simulink model "EMR_WindTurbine_Final"  (R2022b)
settings: Solver=VariableStepAuto  StartTime=0.0  StopTime=10.0  RelTol=1e-3
values from neighbouring files (symbols this model uses):
  b = 15    [Init_Celc.m]
  cmaxfit = -4.70546620480099*(10.^-8)*temp.^4+	3.49662102291610*(10.^-6)*temp.^3 +	0.00209286380926111*temp.^2	-0.0176104377910828*temp+	0.0300191236909972    [Init_Celc.m]
  f = 0.001    [Init_Celc.m]
  J = 0.0015    [Init_Celc.m]
  kr = 1    [Init_Celc.m]
  Ktm = 1.5692    [Init_Celc.m]
  Lr = 0.2395    [Init_Celc.m]
  Ls = 0.256    [Init_Celc.m]
  Msr = 0.236    [Init_Celc.m]
  P = 2    [Init_Celc.m]
  r = 0.75    [Init_Celc.m]
  rho = 1.20    (= 1.2)    [Init_Celc.m]
  Rr = 1.09    [Init_Celc.m]
  Rs = 3.36    [Init_Celc.m]
  s = pi*r.^2    [Init_Celc.m]
  temp = (1:vit_syn/40:vit_syn)    [Init_Celc.m]
  UDC = 620    [Init_Celc.m]
  vf = 230/(2*pi*50)    (= 0.732112738223)    [Init_Celc.m]
settings Model: Creator=habayah  LastModifiedBy=ZinouAb
settings ModelReferenceCC: EnableRefExpFcnMdlSchedulingChecks=on

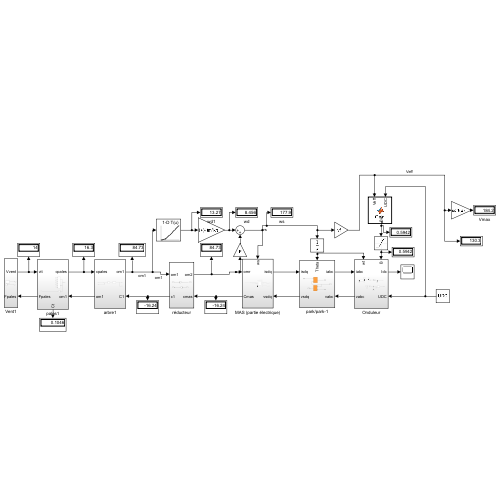
[thumbnail: Simulink's stored preview of the top-level diagram]
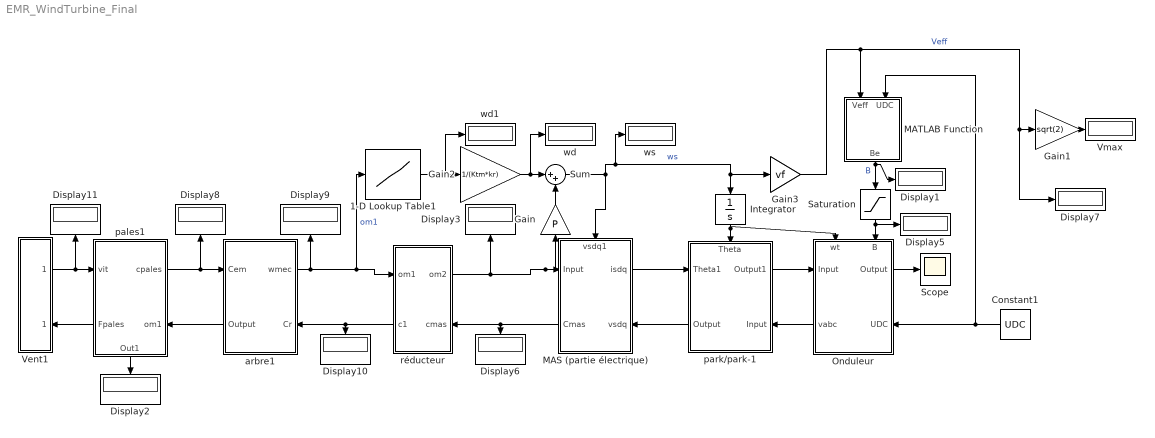
== system EMR_WindTurbine_Final ==
  1-D Lookup Table1 : Lookup_n-D  NumberOfTableDimensions=1  BreakpointsForDimension1=temp  Table=cmaxfit  InternalRulePriority=Speed  RndMeth=Simplest
  Constant1 : Constant  Value=UDC
  Display{1..3,5..11} (10 alike) : Display
  Gain : Gain  Gain=P
  Gain1 : Gain  Gain=sqrt(2)
  Gain2 : Gain  Gain=1/(Ktm*kr)
  Gain3 : Gain  Gain=vf
  Integrator : Integrator
  MAS (partie électrique) : Subsystem
      settings: PortSchema="{\"entries\":[{\"content\":{\"sides\":[{\"content\":{\"connectorIds\":[\"Out2\",\"In1\"]},\"type\":\"ConnectorPlacement.EquallySpacedRectSide\",\"uuid\":\"2ecec5eb-5bb6-4f05-bbbb-1a51ae98f814\"},{\"content\":{\"connectorIds\":[\"In3\",\"Out1\"],\"side\":\"RIGHT\"},\"type\":\"ConnectorPlacement.EquallySpacedRectSide\",\"uuid\":\"ddc3d36f-31b1-43d5-b617-6997f76d08f1\"},{\"content\":{\"connectorIds\":[\"In2\"],\"side\":\"TOP\"},\"type\":\"ConnectorPlacement.EquallySpacedRectSide\",\"uuid\":\"42603242-cda1-4bb2-8cac-1b3409f39577\"}]},\"type\":\"ConnectorPlacement.EquallySpacedConnector\",\"uuid\":\"febb8687-16a8-4638-bd43-9ebf443fd4bd\"}],\"packageUris\":[\"http://schema.mathworks.com/mf0/Connector/R2020b\"],\"version\":\"1.0\"}"
  MATLAB Function : MATLAB Function  TreatAsAtomicUnit=on
  Onduleur : Subsystem
      settings: PortSchema="{\"entries\":[{\"content\":{\"sides\":[{\"content\":{\"connectorIds\":[\"In1\",\"Out2\"]},\"type\":\"ConnectorPlacement.EquallySpacedRectSide\",\"uuid\":\"b96697a1-7390-4a4c-a090-1d4840f94579\"},{\"content\":{\"connectorIds\":[\"Out1\",\"In4\"],\"side\":\"RIGHT\"},\"type\":\"ConnectorPlacement.EquallySpacedRectSide\",\"uuid\":\"06d1d8c6-d481-421b-9786-6ed8bea33fb5\"},{\"content\":{\"connectorIds\":[\"In2\",\"In3\"],\"side\":\"TOP\"},\"type\":\"ConnectorPlacement.EquallySpacedRectSide\",\"uuid\":\"2e081ee8-1238-4450-99c4-3d0e60d3e391\"}]},\"type\":\"ConnectorPlacement.EquallySpacedConnector\",\"uuid\":\"e9990dc2-fc0c-4c65-980c-f90091d8c920\"}],\"packageUris\":[\"http://schema.mathworks.com/mf0/Connector/R2020b\"],\"version\":\"1.0\"}"
  Saturation : Saturate  UpperLimit=1  LowerLimit=0
  Scope : Scope
  Sum : Sum  Inputs=|++
  Vent1 : Subsystem
      settings: PortSchema="{\"entries\":[{\"content\":{\"sides\":[{\"content\":{\"connectorIds\":[]},\"type\":\"ConnectorPlacement.EquallySpacedRectSide\",\"uuid\":\"be9e5db0-62db-41cd-9655-d6d790779573\"},{\"content\":{\"connectorIds\":[\"Out1\",\"In1\"],\"side\":\"RIGHT\"},\"type\":\"ConnectorPlacement.EquallySpacedRectSide\",\"uuid\":\"b5e788b3-1e5f-4899-a162-7a564b67bc63\"},{\"content\":{\"connectorIds\":[],\"side\":\"TOP\"},\"type\":\"ConnectorPlacement.EquallySpacedRectSide\",\"uuid\":\"cac5ef03-1794-4810-a86f-81d9785b0908\"}]},\"type\":\"ConnectorPlacement.EquallySpacedConnector\",\"uuid\":\"fdefeacd-144d-477b-b7c5-141053c244e1\"}],\"packageUris\":[\"http://schema.mathworks.com/mf0/Connector/R2020b\"],\"version\":\"1.0\"}"
  Vmax : Display
  arbre1 : Subsystem
      settings: PortSchema="{\"entries\":[{\"content\":{\"sides\":[{\"content\":{\"connectorIds\":[\"In1\",\"Out2\"]},\"type\":\"ConnectorPlacement.EquallySpacedRectSide\",\"uuid\":\"b8908f99-787f-4ebd-a8c4-361ef654133e\"},{\"content\":{\"connectorIds\":[\"Out1\",\"In2\"],\"side\":\"RIGHT\"},\"type\":\"ConnectorPlacement.EquallySpacedRectSide\",\"uuid\":\"e7049b46-0747-4182-8580-458ffa90f1c3\"},{\"content\":{\"connectorIds\":[],\"side\":\"TOP\"},\"type\":\"ConnectorPlacement.EquallySpacedRectSide\",\"uuid\":\"013bc89f-8670-489b-af07-681a8894793a\"}]},\"type\":\"ConnectorPlacement.EquallySpacedConnector\",\"uuid\":\"dba8a148-0e4d-4308-b676-65e370746724\"}],\"packageUris\":[\"http://schema.mathworks.com/mf0/Connector/R2020b\"],\"version\":\"1.0\"}"
  pales1 : Subsystem
      settings: PortSchema="{\"entries\":[{\"content\":{\"sides\":[{\"content\":{\"connectorIds\":[\"In1\",\"Out3\"]},\"type\":\"ConnectorPlacement.EquallySpacedRectSide\",\"uuid\":\"2ecec5eb-5bb6-4f05-bbbb-1a51ae98f814\"},{\"content\":{\"connectorIds\":[\"Out1\",\"In2\"],\"side\":\"RIGHT\"},\"type\":\"ConnectorPlacement.EquallySpacedRectSide\",\"uuid\":\"ddc3d36f-31b1-43d5-b617-6997f76d08f1\"},{\"content\":{\"connectorIds\":[],\"side\":\"TOP\"},\"type\":\"ConnectorPlacement.EquallySpacedRectSide\",\"uuid\":\"42603242-cda1-4bb2-8cac-1b3409f39577\"},{\"content\":{\"connectorIds\":[\"Out2\"],\"side\":\"BOTTOM\"},\"type\":\"ConnectorPlacement.EquallySpacedRectSide\",\"uuid\":\"35b11503-f988-4bb4-a280-dcf5d49d8570\"}]},\"type\":\"ConnectorPlacement.EquallySpacedConnector\",\"uuid\":\"febb8687-16a8-4638-bd43-9ebf443fd4bd\"}],\"packageUris\":[\"http://schema.mathworks.com/mf0/Connector/R2020b\"],\"version\":\"1.0\"}"
  park/park-1 : Subsystem
      settings: PortSchema="{\"entries\":[{\"content\":{\"sides\":[{\"content\":{\"connectorIds\":[\"In1\",\"Out2\"]},\"type\":\"ConnectorPlacement.EquallySpacedRectSide\",\"uuid\":\"83ad06b1-0178-473a-86b5-0d897bfdf029\"},{\"content\":{\"connectorIds\":[\"Out1\",\"In3\"],\"side\":\"RIGHT\"},\"type\":\"ConnectorPlacement.EquallySpacedRectSide\",\"uuid\":\"370b5efa-4dd6-4b26-a8f3-51e0a3b4d610\"},{\"content\":{\"connectorIds\":[\"In2\"],\"side\":\"TOP\"},\"type\":\"ConnectorPlacement.EquallySpacedRectSide\",\"uuid\":\"4ed8d0b1-afea-41b0-b5a1-8f5ae24d8944\"},{\"content\":{\"connectorIds\":[],\"side\":\"BOTTOM\"},\"type\":\"ConnectorPlacement.EquallySpacedRectSide\",\"uuid\":\"28d6add2-f293-47f7-8dcb-eb46b3627242\"}]},\"type\":\"ConnectorPlacement.EquallySpacedConnector\",\"uuid\":\"0d95acdc-2677-48aa-afd9-0dc380a25251\"}],\"packageUris\":[\"http://schema.mathworks.com/mf0/Connector/R2020b\"],\"version\":\"1.0\"}"
  réducteur : Subsystem
      settings: PortSchema="{\"entries\":[{\"content\":{\"sides\":[{\"content\":{\"connectorIds\":[\"In1\",\"Out2\"]},\"type\":\"ConnectorPlacement.EquallySpacedRectSide\",\"uuid\":\"2ecec5eb-5bb6-4f05-bbbb-1a51ae98f814\"},{\"content\":{\"connectorIds\":[\"Out1\",\"In2\"],\"side\":\"RIGHT\"},\"type\":\"ConnectorPlacement.EquallySpacedRectSide\",\"uuid\":\"ddc3d36f-31b1-43d5-b617-6997f76d08f1\"},{\"content\":{\"connectorIds\":[],\"side\":\"TOP\"},\"type\":\"ConnectorPlacement.EquallySpacedRectSide\",\"uuid\":\"42603242-cda1-4bb2-8cac-1b3409f39577\"}]},\"type\":\"ConnectorPlacement.EquallySpacedConnector\",\"uuid\":\"febb8687-16a8-4638-bd43-9ebf443fd4bd\"}],\"packageUris\":[\"http://schema.mathworks.com/mf0/Connector/R2020b\"],\"version\":\"1.0\"}"
  wd : Display
  wd1 : Display
  ws : Display
  wires:
  réducteur/1(om2) -> Display3/1, MAS (partie électrique)/3(Input), Gain/1
  MAS (partie électrique)/1(Cmas) -> Display6/1, réducteur/2(cmas)
  MAS (partie électrique)/2(isdq) -> park/park-1/1(Theta1)
  park/park-1/2(Output) -> MAS (partie électrique)/1(vsdq)
  Gain/1 -> Sum/2
  Integrator/1 -> Onduleur/2(wt), park/park-1/2(Theta)
  Gain2/1 -> wd/1, Sum/1
  Vent1/1(Out1) -> Display11/1, pales1/1(vit)
  réducteur/2(c1) -> arbre1/2(Cr), Display10/1
  pales1/1(cpales) -> arbre1/1(Cem), Display8/1
  arbre1/1(wmec) -> réducteur/1(om1), 1-D Lookup Table1/1, Display9/1  "om1"
  arbre1/2(Output) -> pales1/2(om1)
  pales1/3(Fpales) -> Vent1/1(In1)
  Sum/1 -> MAS (partie électrique)/2(vsdq1), ws/1, Integrator/1, Gain3/1  "ws"
  Gain1/1 -> Vmax/1
  Saturation/1 -> Onduleur/3(B), Display5/1
  Gain3/1 -> Display7/1, Gain1/1, MATLAB Function/1(Veff)  "Veff"
  MATLAB Function/1(Be) -> Display1/1, Saturation/1  "B"
  Constant1/1 -> Onduleur/4(UDC), MATLAB Function/2(UDC)
  Onduleur/2(vabc) -> park/park-1/3(Input)
  park/park-1/1(Output1) -> Onduleur/1(Input)
  Onduleur/1(Output) -> Scope/1
  pales1/2(Out1) -> Display2/1
  1-D Lookup Table1/1 -> wd1/1, Gain2/1

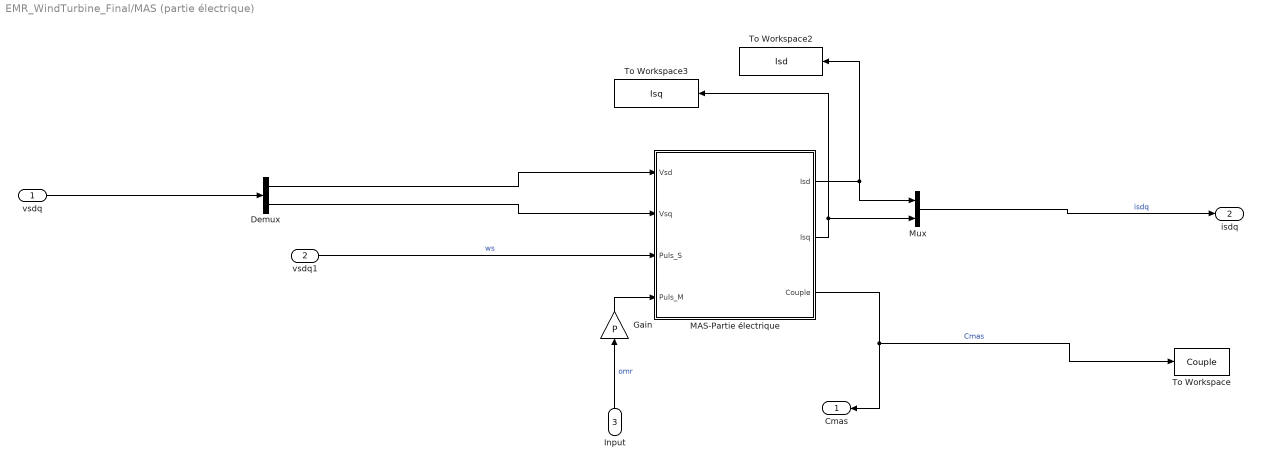
== system EMR_WindTurbine_Final/MAS (partie électrique) ==
  vsdq : Inport
  vsdq1 : Inport  Port=2
  Input : Inport  Port=3
  Demux : Demux  Outputs=2
  Gain : Gain  Gain=P
  MAS-Partie électrique : Subsystem
  Mux : Mux  Inputs=2
  To Workspace : ToWorkspace  VariableName=Couple  SampleTime=-1
      settings: Save2DSignal=2-D array (concatenate along first dimension)
  To Workspace2 : ToWorkspace  VariableName=Isd  SaveFormat=Timeseries  SampleTime=-1
  To Workspace3 : ToWorkspace  VariableName=Isq  SaveFormat=Timeseries  SampleTime=-1
  Cmas : Outport
  isdq : Outport  Port=2
  wires:
  MAS-Partie électrique/2(Isq) -> Mux/2, To Workspace3/1
  MAS-Partie électrique/3(Couple) -> Cmas/1, To Workspace/1  "Cmas"
  Demux/2 -> MAS-Partie électrique/2(Vsq)
  MAS-Partie électrique/1(Isd) -> Mux/1, To Workspace2/1
  Gain/1 -> MAS-Partie électrique/4(Puls_M)
  Input/1 -> Gain/1  "omr"
  Demux/1 -> MAS-Partie électrique/1(Vsd)
  Mux/1 -> isdq/1  "isdq"
  vsdq/1 -> Demux/1
  vsdq1/1 -> MAS-Partie électrique/3(Puls_S)  "ws"

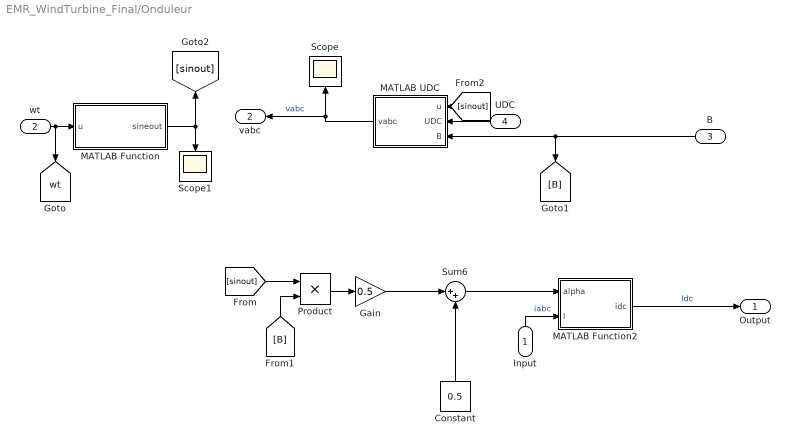
== system EMR_WindTurbine_Final/Onduleur ==
  Input : Inport
  wt : Inport  Port=2
  B : Inport  Port=3
  UDC : Inport  Port=4
  Constant : Constant  Value=0.5
  Gain : Gain  Gain=0.5
  MATLAB Function : MATLAB Function  TreatAsAtomicUnit=on
  MATLAB Function2 : MATLAB Function  TreatAsAtomicUnit=on
  MATLAB UDC : MATLAB Function  TreatAsAtomicUnit=on
  Product : Product
  Scope : Scope
  Scope1 : Scope
  Sum6 : Sum  Inputs=|++
  Output : Outport
  vabc : Outport  Port=2
  tag scope: wt=global
  wires:
  MATLAB Function/1(sineout) -> Scope1/1, [sinout]
  wt/1 -> MATLAB Function/1(u), [wt]
  MATLAB UDC/1(vabc) -> Scope/1, vabc/1  "vabc"
  B/1 -> MATLAB UDC/3(B), [B]
  UDC/1 -> MATLAB UDC/2(UDC)
  [sinout] -> Product/1
  [B] -> Product/2
  Product/1 -> Gain/1
  Sum6/1 -> MATLAB Function2/1(alpha)
  Constant/1 -> Sum6/2
  Input/1 -> MATLAB Function2/2(I)  "iabc"
  MATLAB Function2/1(idc) -> Output/1  "Idc"
  Gain/1 -> Sum6/1
  [sinout] -> MATLAB UDC/1(u)

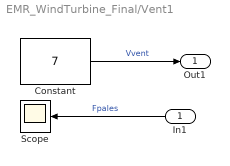
== system EMR_WindTurbine_Final/Vent1 ==
  In1 : Inport
  Constant : Constant  Value=7
  Scope : Scope
  Out1 : Outport
  wires:
  In1/1 -> Scope/1  "Fpales"
  Constant/1 -> Out1/1  "Vvent"

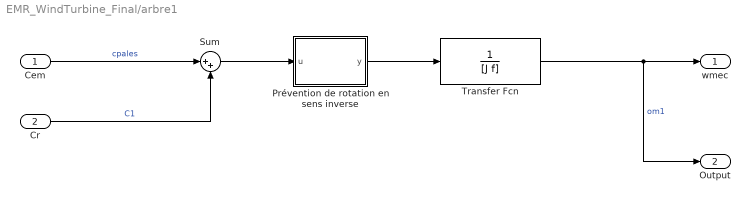
== system EMR_WindTurbine_Final/arbre1 ==
  Cem : Inport
  Cr : Inport  Port=2
  Prévention de rotation en sens inverse : MATLAB Function  TreatAsAtomicUnit=on
  Sum : Sum  Inputs=|++
  Transfer Fcn : TransferFcn  Denominator=[J f]
  wmec : Outport
  Output : Outport  Port=2
  wires:
  Cem/1 -> Sum/1  "cpales"
  Sum/1 -> Prévention de rotation en sens inverse/1(u)
  Cr/1 -> Sum/2  "C1"
  Transfer Fcn/1 -> Output/1, wmec/1  "om1"
  Prévention de rotation en sens inverse/1(y) -> Transfer Fcn/1

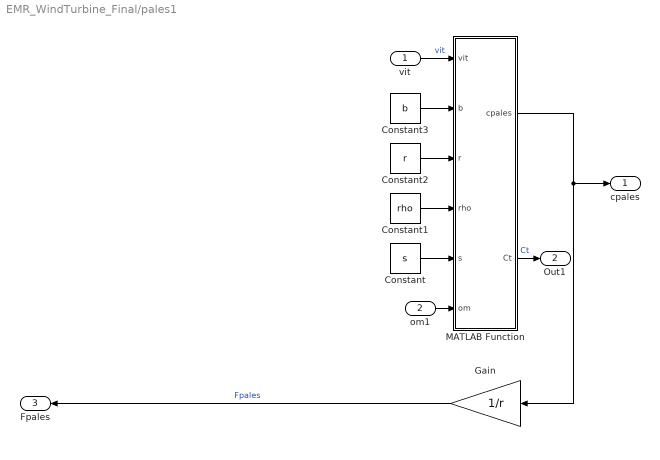
== system EMR_WindTurbine_Final/pales1 ==
  vit : Inport
  om1 : Inport  Port=2
  Constant : Constant  Value=s
  Constant1 : Constant  Value=rho
  Constant2 : Constant  Value=r
  Constant3 : Constant  Value=b
  Gain : Gain  Gain=1/r
  MATLAB Function : MATLAB Function  TreatAsAtomicUnit=on
  cpales : Outport
  Out1 : Outport  Port=2
  Fpales : Outport  Port=3
  wires:
  vit/1 -> MATLAB Function/1(vit)  "vit"
  om1/1 -> MATLAB Function/6(om)
  Constant2/1 -> MATLAB Function/3(r)
  MATLAB Function/1(cpales) -> Gain/1, cpales/1
  Gain/1 -> Fpales/1  "Fpales"
  Constant/1 -> MATLAB Function/5(s)
  Constant1/1 -> MATLAB Function/4(rho)
  Constant3/1 -> MATLAB Function/2(b)
  MATLAB Function/2(Ct) -> Out1/1  "Ct"

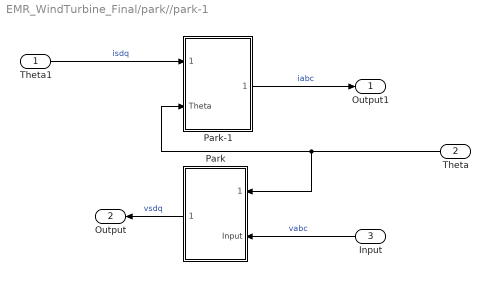
== system EMR_WindTurbine_Final/park//park-1 ==
  Theta1 : Inport
  Theta : Inport  Port=2
  Input : Inport  Port=3
  Park : Subsystem
  Park-1 : Subsystem
  Output1 : Outport
  Output : Outport  Port=2
  wires:
  Theta/1 -> Park/1(Theta), Park-1/2(Theta)
  Theta1/1 -> Park-1/1(Theta1)  "isdq"
  Input/1 -> Park/2(Input)  "vabc"
  Park/1(Output) -> Output/1  "vsdq"
  Park-1/1(Output) -> Output1/1  "iabc"

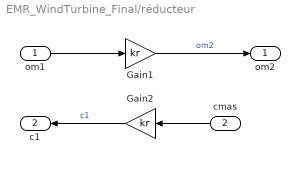
== system EMR_WindTurbine_Final/réducteur ==
  om1 : Inport
  cmas : Inport  Port=2
  Gain1 : Gain  Gain=kr
  Gain2 : Gain  Gain=kr
  om2 : Outport
  c1 : Outport  Port=2
  wires:
  om1/1 -> Gain1/1
  cmas/1 -> Gain2/1
  Gain2/1 -> c1/1  "c1"
  Gain1/1 -> om2/1  "om2"

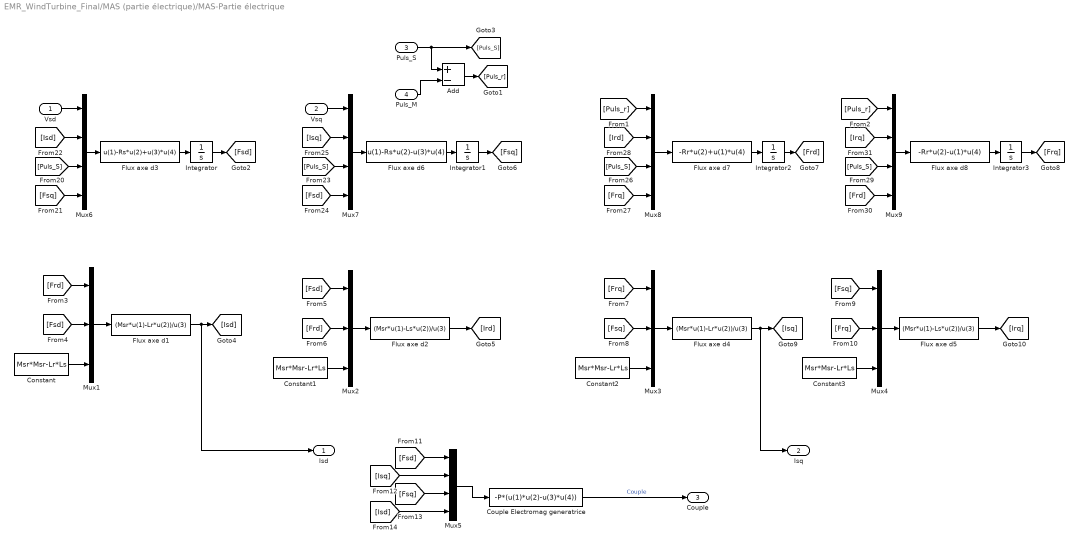
== system EMR_WindTurbine_Final/MAS (partie électrique)/MAS-Partie électrique ==
  Vsd : Inport
  Vsq : Inport  Port=2
  Puls_S : Inport  Port=3
  Puls_M : Inport  Port=4
  Add : Sum  Inputs=+-
  Constant{,1..3} (4 alike) : Constant  Value=Msr*Msr-Lr*Ls
  Couple Electromag generatrice : Fcn  Expr=-P*(u(1)*u(2)-u(3)*u(4))
  Flux axe d1 : Fcn  Expr=(Msr*u(1)-Lr*u(2))/u(3)
  Flux axe d2 : Fcn  Expr=(Msr*u(1)-Ls*u(2))/u(3)
  Flux axe d3 : Fcn  Expr=u(1)-Rs*u(2)+u(3)*u(4)
  Flux axe d4 : Fcn  Expr=(Msr*u(1)-Lr*u(2))/u(3)
  Flux axe d5 : Fcn  Expr=(Msr*u(1)-Ls*u(2))/u(3)
  Flux axe d6 : Fcn  Expr=u(1)-Rs*u(2)-u(3)*u(4)
  Flux axe d7 : Fcn  Expr=-Rr*u(2)+u(1)*u(4)
  Flux axe d8 : Fcn  Expr=-Rr*u(2)-u(1)*u(4)
  Integrator{,1..3} (4 alike) : Integrator
  Mux{1..4} (4 alike) : Mux  Inputs=3
  Mux{5..9} (5 alike) : Mux
  Isd : Outport
  Isq : Outport  Port=2
  Couple : Outport  Port=3
  wires:
  Puls_S/1 -> Add/1, [Puls_S]
  Mux6/1 -> Flux axe d3/1
  Vsd/1 -> Mux6/1
  [Isd] -> Mux6/2
  [Puls_S] -> Mux6/3
  [Fsq] -> Mux6/4
  Flux axe d3/1 -> Integrator/1
  Integrator/1 -> [Fsd]
  Mux7/1 -> Flux axe d6/1
  Vsq/1 -> Mux7/1
  [Isq] -> Mux7/2
  [Puls_S] -> Mux7/3
  [Fsd] -> Mux7/4
  Flux axe d6/1 -> Integrator1/1
  Integrator1/1 -> [Fsq]
  Mux8/1 -> Flux axe d7/1
  [Ird] -> Mux8/2
  [Puls_S] -> Mux8/3
  [Frq] -> Mux8/4
  Flux axe d7/1 -> Integrator2/1
  Integrator2/1 -> [Frd]
  Mux9/1 -> Flux axe d8/1
  [Puls_r] -> Mux8/1
  [Irq] -> Mux9/2
  [Puls_S] -> Mux9/3
  [Frd] -> Mux9/4
  Flux axe d8/1 -> Integrator3/1
  Integrator3/1 -> [Frq]
  [Puls_r] -> Mux9/1
  [Frd] -> Mux1/1
  [Fsd] -> Mux1/2
  Mux1/1 -> Flux axe d1/1
  Constant/1 -> Mux1/3
  Flux axe d1/1 -> Isd/1, [Isd]
  [Fsd] -> Mux2/1
  [Frd] -> Mux2/2
  Mux2/1 -> Flux axe d2/1
  Constant1/1 -> Mux2/3
  Flux axe d2/1 -> [Ird]
  [Frq] -> Mux3/1
  [Fsq] -> Mux3/2
  Mux3/1 -> Flux axe d4/1
  Constant2/1 -> Mux3/3
  Flux axe d4/1 -> Isq/1, [Isq]
  [Fsq] -> Mux4/1
  [Frq] -> Mux4/2
  Mux4/1 -> Flux axe d5/1
  Constant3/1 -> Mux4/3
  Flux axe d5/1 -> [Irq]
  Mux5/1 -> Couple Electromag generatrice/1
  Couple Electromag generatrice/1 -> Couple/1  "Couple"
  [Isd] -> Mux5/4
  [Fsd] -> Mux5/1
  [Isq] -> Mux5/2
  [Fsq] -> Mux5/3
  Puls_M/1 -> Add/2
  Add/1 -> [Puls_r]

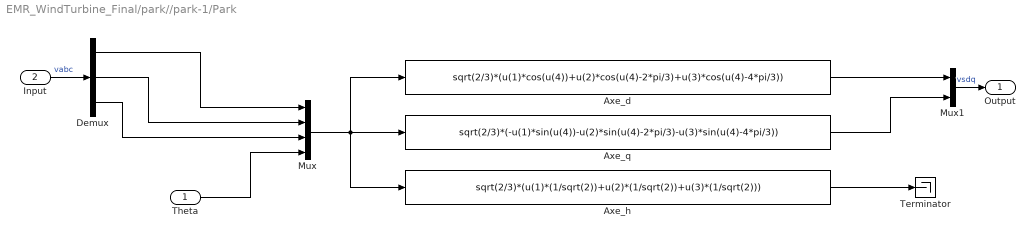
== system EMR_WindTurbine_Final/park//park-1/Park ==
  Theta : Inport
  Input : Inport  Port=2
  " Axe_h" : Fcn  Expr=sqrt(2/3)*(u(1)*(1/sqrt(2))+u(2)*(1/sqrt(2))+u(3)*(1/sqrt(2)))
  " Axe_q" : Fcn  Expr=sqrt(2/3)*(-u(1)*sin(u(4))-u(2)*sin(u(4)-2*pi/3)-u(3)*sin(u(4)-4*pi/3))
  Axe_d : Fcn  Expr=sqrt(2/3)*(u(1)*cos(u(4))+u(2)*cos(u(4)-2*pi/3)+u(3)*cos(u(4)-4*pi/3))
  Demux : Demux  Outputs=3
  Mux : Mux
  Mux1 : Mux  Inputs=2
  Terminator : Terminator
  Output : Outport
  wires:
  Demux/1 -> Mux/1
  Demux/2 -> Mux/2
  Demux/3 -> Mux/3
  Theta/1 -> Mux/4
  Mux/1 -> " Axe_q"/1, " Axe_h"/1, Axe_d/1
  " Axe_h"/1 -> Terminator/1
  " Axe_q"/1 -> Mux1/2
  Axe_d/1 -> Mux1/1
  Input/1 -> Demux/1  "vabc"
  Mux1/1 -> Output/1  "vsdq"

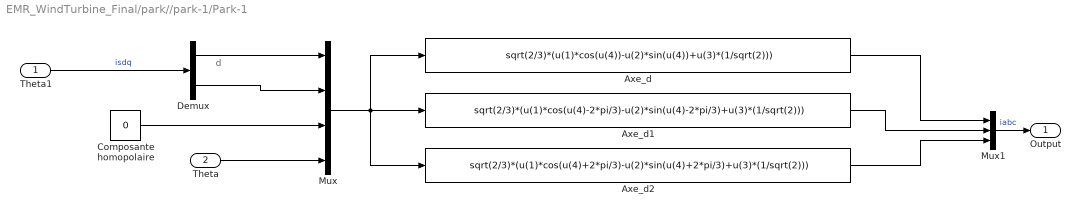
== system EMR_WindTurbine_Final/park//park-1/Park-1 ==
  note: d
  Theta1 : Inport
  Theta : Inport  Port=2
  Axe_d : Fcn  Expr=sqrt(2/3)*(u(1)*cos(u(4))-u(2)*sin(u(4))+u(3)*(1/sqrt(2)))
  Axe_d1 : Fcn  Expr=sqrt(2/3)*(u(1)*cos(u(4)-2*pi/3)-u(2)*sin(u(4)-2*pi/3)+u(3)*(1/sqrt(2)))
  Axe_d2 : Fcn  Expr=sqrt(2/3)*(u(1)*cos(u(4)+2*pi/3)-u(2)*sin(u(4)+2*pi/3)+u(3)*(1/sqrt(2)))
  Composante homopolaire : Constant  Value=0
  Demux : Demux  Outputs=2
  Mux : Mux
  Mux1 : Mux  Inputs=3
  Output : Outport
  wires:
  Demux/1 -> Mux/1
  Demux/2 -> Mux/2
  Mux/1 -> Axe_d1/1, Axe_d2/1, Axe_d/1
  Axe_d2/1 -> Mux1/3
  Axe_d1/1 -> Mux1/2
  Axe_d/1 -> Mux1/1
  Theta/1 -> Mux/4
  Composante homopolaire/1 -> Mux/3
  Theta1/1 -> Demux/1  "isdq"
  Mux1/1 -> Output/1  "iabc"

== matlab function EMR_WindTurbine_Final/Onduleur/MATLAB Function2 ==
  data: alpha input; idc output; I input
function idc = idcfcn(alpha,I)

idc = 0.5*(alpha)'*I;

== matlab function EMR_WindTurbine_Final/Onduleur/MATLAB Function ==
  data: u input; sineout output
function sineout = Sinegenerator(u)

y1 = sin(u);
y2 = sin(u-2*pi/3);
y3 = sin(u+2*pi/3);

sineout=[y1; y2;y3];

== matlab function EMR_WindTurbine_Final/arbre1/Prévention de rotation en sens inverse ==
  data: u input; y output
function y = fcn(u)
if u>0
    y=u;
else
    y=0;
end

== matlab function EMR_WindTurbine_Final/MATLAB Function ==
  data: Veff input; UDC input; Be output
function Be = Gain(Veff,UDC)

Be =Veff* 2*sqrt(2)/UDC;

== matlab function EMR_WindTurbine_Final/pales1/MATLAB Function ==
  data: vit input; b input; cpales output; r input; rho input; s input; om input; Ct output
function [cpales,Ct] = fcn(vit,b,r,rho,s,om)

    lamb=r*om/vit;
  
    if lamb==0    % Pour éviter d'avoir une division par zero par la suite
        lamb=0.001;
    end
        lamb1=1/((1/(lamb+0.089*b))-(0.035/(b^3+1)));
        Cp=0.5*(116/lamb1-0.4*(b-5))*exp(-16.5/lamb1);
        Ct=Cp/lamb;
        
        if Ct<=0
            Ct=0.01;
        end

        cpales=0.5*rho*Ct*r*s*vit^2;





end

== matlab function EMR_WindTurbine_Final/Onduleur/MATLAB UDC ==
  data: u input; UDC input; vabc output; B input
function vabc = gain(u,UDC,B)


vabc =0.5*UDC*B.*u;
